simulink model "Lab11"  (R2017a)
settings: Solver=VariableStepAuto  StartTime=0.0  StopTime=0.01  MaxStep=0.000010001  MinStep=0.00001  RelTol=1e-6
undefined symbols (not defined in the file): Cp, Fv, Kd, Kf, Ko, Ku, Kv, Kx, m, Tu, U
settings Model: Creator=User  LastModifiedBy=User

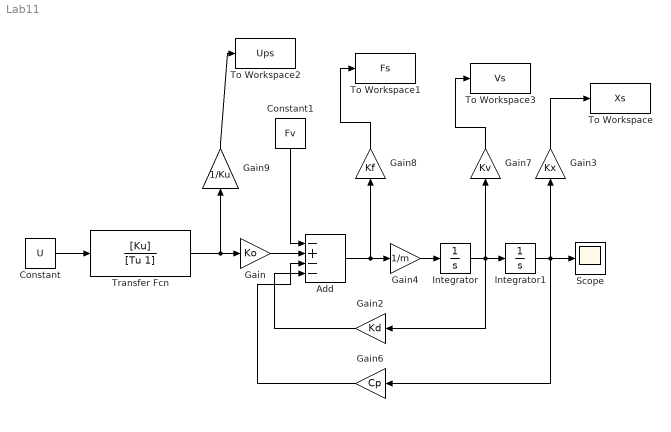
== system Lab11 ==
  Add : Sum  Inputs=-+--
  Constant : Constant  Value=U
  Constant1 : Constant  Value=Fv
  Gain : Gain  Gain=Ko
  Gain2 : Gain  Gain=Kd
  Gain3 : Gain  Gain=Kx
  Gain4 : Gain  Gain=1/m
  Gain6 : Gain  Gain=Cp
  Gain7 : Gain  Gain=Kv
  Gain8 : Gain  Gain=Kf
  Gain9 : Gain  Gain=1/Ku
  Integrator : Integrator
  Integrator1 : Integrator
  Scope : Scope
  To Workspace : ToWorkspace  VariableName=Xs  SampleTime=-1
  To Workspace1 : ToWorkspace  VariableName=Fs  SampleTime=-1
  To Workspace2 : ToWorkspace  VariableName=Ups  SampleTime=-1
  To Workspace3 : ToWorkspace  VariableName=Vs  SampleTime=-1
  Transfer Fcn : TransferFcn  Numerator=[Ku]  Denominator=[Tu 1]
  wires:
  Constant/1 -> Transfer Fcn/1
  Transfer Fcn/1 -> Gain9/1, Gain/1
  Gain/1 -> Add/2
  Add/1 -> Gain8/1, Gain4/1
  Gain4/1 -> Integrator/1
  Integrator/1 -> Gain7/1, Integrator1/1, Gain2/1
  Constant1/1 -> Add/1
  Gain2/1 -> Add/4
  Integrator1/1 -> Gain6/1, Scope/1, Gain3/1
  Gain6/1 -> Add/3
  Gain9/1 -> To Workspace2/1
  Gain8/1 -> To Workspace1/1
  Gain7/1 -> To Workspace3/1
  Gain3/1 -> To Workspace/1
